simulink library "sm_car_4post_lib"  (R2021b)
settings: Solver=VariableStepAuto  StartTime=0.0  StopTime=10.0  RelTol=1e-3
values from neighbouring files (symbols this model uses):
  Init = struct    [sm_car_4post_init_data.m]
  N = 100    [sm_extr_data_cam_roller_curve.m]
  s = sin(q)    [sm_extr_data_cam_roller_curve.m]
  Vehicle = Vehicle_03    [sm_car_4post_gen_op.m]    (also in sm_car_4post_testrig_plot2testall.m)
undefined symbols (not defined in the file or in its folder): clr_upr, hp_in_f_ua, hp_in_r_ua, hp_la_out, hp_ua_out, LAc, LAf, LAr, opc_upr, radius_upr, rhs_hp, sm_car_4post_platform, smcar_param, UAc, UAf, UAr, X, Y, Z
libraries: sm_lib x234, $bdroot x71, fl_lib x24, nesl_utility x21, simulink x3
(part 2 of 11)

== system sm_car_4post_lib/Shafts CVCV ==
  CVCV : Subsystem  VariantControl=CVCV  mask(Shafts with Constant Velocity Joints){popup_leftRight=Right, drv_sha_hp_transaxle_l=Shaft.Transaxle.sTransaxle.Value, drv_sha_transax_m=Shaft.Transaxle.m.Value, drv_sha_drvsh_m=Shaft.Driveshaft.m.Value, drv_sha_axle_m=Shaft.Axle.m.Value, clr_drv_sha_hp=smcar_param.hp.clr, opc_drv_sha_hp=smcar_param.hp.opc, rad_drv_sha_hp=smcar_param.hp.rad, clr_drv_sha_jnt=smcar_param.red, opc_drv_sha_jnt=smcar_param.part.opc, rad_drv_sha_jnt=0.03, clr_drv_sha_transax=smcar_param.gray, opc_drv_sha_transax=smcar_param.part.opc, rad_drv_sha_transax=0.025, clr_drv_sha_drvsh=smcar_param.gray, opc_drv_sha_drvsh=smcar_param.part.opc, rad_drv_sha_drvsh=0.025, clr_drv_sha_axle=smcar_param.gray, opc_drv_sha_axle=smcar_param.part.opc, rad_drv_sha_axle=0.025, len_drv_sha_transax=Shaft.Transaxle.l.Value, len_drv_sha_drvsh=Shaft.Driveshaft.l.Value, len_drv_sha_axle=Shaft.Axle.l.Value}
      mask prompts: popup_leftRight "Left/Right"; drv_sha_hp_transaxle_l "Transaxle HP [xyz] (m)"; drv_sha_transax_m "Transaxle Mass (kg)"; drv_sha_drvsh_m "Driveshaft Mass (kg)"; drv_sha_axle_m "Axle Mass (kg)"; len_drv_sha_transax "Transaxle Length (m)"; len_drv_sha_drvsh "Driveshaft Length (m)"; len_drv_sha_axle "Axle Length (m)"
      mask help: Driveshaft with Constant Velocity Joints at either end.
      mask init:
      | sm_car_4post_lib_setLeftRight(gcb,'none');
      mask TypeOptions popup_leftRight: Left | Right
      mask TypeOptions drv_sha_hp_transaxle_l:
      | Transform
      | HP Transaxle/TranslationCartesianOffset
      mask TypeOptions drv_sha_transax_m: Transaxle/shaft_m
      mask TypeOptions drv_sha_drvsh_m: Driveshaft/shaft_m
      mask TypeOptions drv_sha_axle_m: Axle/shaft_m
      mask TypeOptions clr_drv_sha_hp:
      | Vis HP
      | Transaxle/GraphicDiffuseColor
      mask TypeOptions opc_drv_sha_hp:
      | Vis HP
      | Transaxle/GraphicOpacity
      mask TypeOptions rad_drv_sha_hp:
      | Vis HP
      | Transaxle/SphereRadius
      mask TypeOptions clr_drv_sha_jnt:
      | Vis
      | CV Joint
      | Inboard/GraphicDiffuseColor | Vis
      | CV Joint
      | Outboard/GraphicDiffuseColor
      mask TypeOptions opc_drv_sha_jnt:
      | Vis
      | CV Joint
      | Inboard/GraphicOpacity | Vis
      | CV Joint
      | Outboard/GraphicOpacity
      mask TypeOptions rad_drv_sha_jnt:
      | Vis
      | CV Joint
      | Inboard/SphereRadius | Vis
      | CV Joint
      | Outboard/SphereRadius
      mask TypeOptions clr_drv_sha_transax: Transaxle/clr_shaft
      mask TypeOptions opc_drv_sha_transax: Transaxle/opc_shaft
      mask TypeOptions rad_drv_sha_transax: Transaxle/rad_shaft
      mask TypeOptions clr_drv_sha_drvsh: Driveshaft/clr_shaft
      mask TypeOptions opc_drv_sha_drvsh: Driveshaft/opc_shaft
      mask TypeOptions rad_drv_sha_drvsh: Driveshaft/rad_shaft
      mask TypeOptions clr_drv_sha_axle: Axle/clr_shaft
      mask TypeOptions opc_drv_sha_axle: Axle/opc_shaft
      mask TypeOptions rad_drv_sha_axle: Axle/rad_shaft
      mask TypeOptions len_drv_sha_transax: Transaxle/len_shaft
      mask TypeOptions len_drv_sha_drvsh: Driveshaft/len_shaft
      mask TypeOptions len_drv_sha_axle: Axle/len_shaft
      mask DialogControl cont_vis_drv_sha Prompt: Visualization
      mask DialogControl text_vis_drv_sha_clr Prompt: Color [RGB]
      mask DialogControl text_vis_drv_sha_opc Prompt: Opac. (0-1)
      mask DialogControl text_vis_drv_sha_rad Prompt: Radius (m)
      mask DialogControl text_vis_drv_sha_hp Prompt: Hardpoints
      mask DialogControl text_vis_drv_sha_joints Prompt: Joints
      mask DialogControl text_vis_drv_sha_transax Prompt: Transaxle
      mask DialogControl text_vis_drv_sha_drvsh Prompt: Driveshaft
      mask DialogControl text_vis_axle_drvsh Prompt: Axle
  F : PMIOPort  Side=Right
  P : PMIOPort  Port=2  Side=Right
  B : PMIOPort  Port=3  Side=Left
  connections:
  CVCV/RConn2 -- P/RConn1
  CVCV/RConn1 -- F/RConn1
  CVCV/LConn1 -- B/RConn1

== system sm_car_4post_lib/Shafts None ==
  None : Subsystem  VariantControl=None
  F : PMIOPort  Side=Right
  P : PMIOPort  Port=2  Side=Right
  B : PMIOPort  Port=3  Side=Left
  connections:
  None/LConn1 -- B/RConn1
  None/RConn1 -- F/RConn1
  None/RConn2 -- P/RConn1

== system sm_car_4post_lib/Sine Input ==
  Clock : Clock
  Constant : Constant  Value=wave_period*num_periods+wave_delay
  Gain : Gain  Gain=wave_amplitude
  GreaterThan : RelationalOperator  Operator=<  OutDataTypeStr=boolean  RndMeth=Simplest
  Product : Product
  Ramp : simulink/Sources/Ramp  slope=2*pi/wave_period  start=wave_delay  InitialOutput=0
  Sine Wave Function : Sin  TimeSource=Use external signal  SampleTime=0
  Out1 : Outport  VectorParamsAs1DForOutWhenUnconnected=off
  wires:
  Sine Wave Function/1 -> Gain/1
  Constant/1 -> GreaterThan/2
  Clock/1 -> GreaterThan/1
  GreaterThan/1 -> Product/2
  Gain/1 -> Product/1
  Ramp/1 -> Sine Wave Function/1
  Product/1 -> Out1/1

== system sm_car_4post_lib/Spring ==
  Ctrl : Inport
  Linear : Subsystem  VariantControl=Linear  mask(Linear Spring){spr_def0=Spring.xPreload.Value, spr_k=Spring.K.Value, spr_hp_top=Spring.sTop.Value, spr_hp_bot=Spring.sBottom.Value}
      mask prompts: spr_def0 "Spr. Preload (m)"; spr_k "Spring Rate (N/m)"; spr_hp_top "HP Top [xyz] (m)"; spr_hp_bot "HP Bottom [xyz] (m)"
      mask help: Spring with linear behavior with measurements.
      mask init:
      | spr_len0 = norm(spr_hp_top-spr_hp_bot);
  R : PMIOPort  Side=Left
  C : PMIOPort  Port=2  Side=Right
  meas : Outport  VectorParamsAs1DForOutWhenUnconnected=off
  wires:
  Ctrl/1 -> Linear/1(Ctrl)
  Linear/1(meas) -> meas/1
  connections:
  Linear/RConn1 -- C/RConn1
  Linear/LConn1 -- R/RConn1

== system sm_car_4post_lib/Suspension and Steering ==
  CtrlBus : Inport
  DrvBus : Inport  Port=2
  Linkage : Subsystem  VariantControl=Linkage
  AxleL : PMIOPort  Side=Left
  Ref : PMIOPort  Port=2  Side=Right
  AxleR : PMIOPort  Port=3  Side=Right
  BrkL : PMIOPort  Port=4  Side=Left
  BrkR : PMIOPort  Port=5  Side=Right
  SprL : PMIOPort  Port=6  Side=Left
  SprR : PMIOPort  Port=7  Side=Right
  DmpL : PMIOPort  Port=8  Side=Left
  DmpR : PMIOPort  Port=9  Side=Right
  OutBus : Outport  VectorParamsAs1DForOutWhenUnconnected=off
  wires:
  CtrlBus/1 -> Linkage/1(CtrlBus)
  Linkage/1(OutBus) -> OutBus/1
  DrvBus/1 -> Linkage/2(DrvBus)
  connections:
  Linkage/LConn1 -- AxleL/RConn1
  Linkage/RConn1 -- Ref/RConn1
  Linkage/RConn4 -- SprR/RConn1
  Linkage/RConn5 -- DmpR/RConn1
  Linkage/LConn2 -- BrkL/RConn1
  Linkage/LConn3 -- SprL/RConn1
  Linkage/RConn2 -- AxleR/RConn1
  Linkage/LConn4 -- DmpL/RConn1
  Linkage/RConn3 -- BrkR/RConn1

== system sm_car_4post_lib/Utilities ==
  Camera Frames : Subsystem
      mask Display: disp('Cam')
  Cylinder Between Two Points : Subsystem  mask{hp_b=hp_la_out.*rhs_hp, hp_f=hp_ua_out.*rhs_hp, Mass=0, clr_solid=clr_upr*0+[0.2 0.4 0.6], opc_solid=opc_upr*0.5, rad_solid=radius_upr*1.5}
      mask prompts: hp_b "Hardpoint at B [xyz] (m)"; hp_f "Hardpoint at F [xyz] (m)"; Mass "Mass (kg)"; clr_solid "Color [RGB]"; opc_solid "Opacity (0-1)"; rad_solid "Radius (m)"
      mask TypeOptions Mass: Solid/Mass
      mask TypeOptions clr_solid: Solid/GraphicDiffuseColor
      mask TypeOptions opc_solid: Solid/GraphicOpacity
      mask TypeOptions rad_solid: Solid/CylinderRadius
      mask DialogControl cont_vis Prompt: Visualization
      mask Display: image(fullfile(matlabroot,'toolbox','physmod','sm','smdemos','car_4post_testrig','images','sm_car_4post_cylinder_two_points.png'))
  Primitive Bushing : Subsystem
      mask Display: image(fullfile(matlabroot,'toolbox','physmod','sm','smdemos','car_4post_testrig','images','sm_car_4post_primitive_bushing.png'));
  Primitive Gimbal : Subsystem
      mask Display: image(fullfile(matlabroot,'toolbox','physmod','sm','smdemos','car_4post_testrig','images','sm_car_4post_primitive_gimbal.png'))
  Terminator : Subsystem
  Transform Align Axis Two Points : Subsystem  mask(Transform Align Axis Two Points){hp_b=[1 1 0], hp_t=[4 5 0], popup_f_axis=+X}
      mask prompts: hp_b "Location of B [xyz] (m)"; hp_t "Target for Frame Axis [xyz] (m)"; popup_f_axis "Axis of F Frame to Aim at Target"
      mask help: Transforms a frame to aim a selected axis at a target point. Both points must be defined relative to the same reference frame.
      mask init:
      | switch popup_f_axis
      |     case 1, vec = [ 1  0  0];
      |     case 2, vec = [ 0  1  0];
      |     case 3, vec = [ 0  0  1];
      |     case 4, vec = [-1  0  0];
      |     case 5, vec = [ 0 -1  0];
      |     case 6, vec = [ 0  0 -1];
      | end
      | 
      | uvec_bt = (hp_t-hp_b)/norm(hp_t-hp_b);
      | rotaxis = cross(vec,uvec_bt);
      | 
      | if (norm(rotaxis)==0)
      |     if (uvec_bt==0)            % hps collocated
      |         rotangle = 0; 
      |     elseif ((uvec_bt+vec)==0)  % vectors antiparallel    
      |         rotangle = pi;
      |         rotaxis = circshift(vec,1);
      |     else                       % vectors parallel
      |         rotangle = 0;          
      |     end
      | else
      |     rotangle = acos(dot(vec,uvec_bt));
      |     %rotangle = acos(dot(vec,(hp_t-hp_b)/norm((hp_t-hp_b))))
      | end
      mask TypeOptions popup_f_axis: +X | +Y | +Z | -X | -Y | -Z
      mask Display: image(fullfile(matlabroot,'toolbox','physmod','sm','smdemos','car_4post_testrig','images','sm_car_4post_transform_align_axis_two_points.png'))
  Universal Two HP : Subsystem  mask{popup_leftRight=Left, hp_f=hp_in_f_ua, hp_r=hp_in_r_ua}
      mask prompts: popup_leftRight "Left/Right"; hp_f "HP Front [xyz] (m)"; hp_r "HP Rear [xyz] (m)"
      mask init:
      | if(popup_leftRight == 1)
      |     rhs_y = 1;
      | elseif(popup_leftRight == 2)
      |     rhs_y = -1;
      | end
      | 
      | rhs_hp = [1 rhs_y 1];
      mask TypeOptions popup_leftRight: Left | Right
      mask Display: image(fullfile(matlabroot,'toolbox','physmod','sm','smdemos','car_4post_testrig','images','sm_car_4post_variant_universal.png'));

== system sm_car_4post_lib/Wheel ==
  RdBus : Inport
  Post : Subsystem  VariantControl=MFEval  mask{popup_leftRight=Left, platform=sm_car_4post_platform, clr_tyre=[0.5 0.5 0.5], opc_tyre=1, clr_rim=[0.8 0.8 0.8], opc_rim=0.5}
      mask prompts: popup_leftRight "Left/Right"; platform "Platform Data"
      mask init:
      | if(popup_leftRight == 1)
      |     set_param([gcb '/Tire Body'],'popup_leftRight','Left');
      |     rhs_whl = [1 1 1];
      | elseif(popup_leftRight == 2)
      |     set_param([gcb '/Tire Body'],'popup_leftRight','Right');
      |     rhs_whl = [1 -1 1];
      | end
      mask TypeOptions popup_leftRight: Left | Right
      mask TypeOptions clr_tyre: Tire Body/clr_tyre
      mask TypeOptions opc_tyre: Tire Body/opc_tyre
      mask TypeOptions clr_rim: Tire Body/clr_rim
      mask TypeOptions opc_rim: Tire Body/opc_rim
      mask DialogControl cont_tire_mfeval Prompt: Platform
      mask DialogControl cont_vis Prompt: Visualization
      mask DialogControl text_vis_clr Prompt: Color [RGB]
      mask DialogControl text_vis_opc Prompt: Opacity (0-1)
      mask DialogControl text_tyre Prompt: Tyre
      mask DialogControl text_rim Prompt: Rim
  B : PMIOPort  Side=Right
  C : PMIOPort  Port=2  Side=Left
  Out : Outport  VectorParamsAs1DForOutWhenUnconnected=off
  wires:
  RdBus/1 -> Post/1(RdBus)
  Post/1(Out) -> Out/1
  connections:
  Post/LConn1 -- C/RConn1
  Post/RConn1 -- B/RConn1

== system sm_car_4post_lib/Damper/Linear ==
  note: Sensing
  Ctrl : Inport
  Bumpstop : fl_lib/Mechanical/Translational Elements/Translational Hard Stop  upper_bnd=bs_lim_upper m  lower_bnd=bs_lim_lower m  stiff_up=bs_k_upper N/m  stiff_low=bs_k_lower N/m  D_up=bs_b_upper N/(m/s)  D_low=bs_b_lower N/(m/s)  model=1  transition=bs_region m  v_specify=off  v_priority=None  v=0 m/s  v_nominal_specify=off  v_nominal_unit=m/s  v_nominal_value=1  f_specify=off  f_priority=None  f=0 N  f_nominal_specify=off  f_nominal_unit=N  f_nominal_value=1  x_specify=off  x_priority=High  x=0 m  x_nominal_specify=off  x_nominal_unit=m  x_nominal_value=1
  Damper : fl_lib/Mechanical/Translational Elements/Translational Damper  D=dam_b N/(m/s)  v_specify=off  v_priority=None  v=0 m/s  v_nominal_specify=off  v_nominal_unit=m/s  v_nominal_value=1  f_specify=off  f_priority=None  f=0 N  f_nominal_specify=off  f_nominal_unit=N  f_nominal_value=1
  Force Bumpstop : fl_lib/Mechanical/Mechanical Sensors/Ideal Force Sensor
  Force Damper : fl_lib/Mechanical/Mechanical Sensors/Ideal Force Sensor
  Motion Damper : fl_lib/Mechanical/Mechanical Sensors/Ideal Translational Motion Sensor  offset=dam_x0 m
  PS-Simulink Converter : nesl_utility/PS-Simulink Converter  PhysicalDomain=network_engine_domain  SubClassName=ps_output  LeftPortType=input  RightPortType=output  PseudoPeriodic=off  Frequencies=[]  Unit=N  AffineConversion=off
      settings: SourceProductBaseCode=PW,SS
  PS-Simulink Converter1 : nesl_utility/PS-Simulink Converter  PhysicalDomain=network_engine_domain  SubClassName=ps_output  LeftPortType=input  RightPortType=output  PseudoPeriodic=off  Frequencies=[]  Unit=N  AffineConversion=off
      settings: SourceProductBaseCode=PW,SS
  PS-Simulink Converter2 : nesl_utility/PS-Simulink Converter  PhysicalDomain=network_engine_domain  SubClassName=ps_output  LeftPortType=input  RightPortType=output  PseudoPeriodic=off  Frequencies=[]  Unit=m/s  AffineConversion=off
      settings: SourceProductBaseCode=PW,SS
  PS-Simulink Converter3 : nesl_utility/PS-Simulink Converter  PhysicalDomain=network_engine_domain  SubClassName=ps_output  LeftPortType=input  RightPortType=output  PseudoPeriodic=off  Frequencies=[]  Unit=m  AffineConversion=off
      settings: SourceProductBaseCode=PW,SS
  Terminator : Terminator
  R : PMIOPort  Side=Left
  C : PMIOPort  Port=2  Side=Right
  Out Bus Element : Outport  VectorParamsAs1DForOutWhenUnconnected=off  PortName=meas  Element=FDamper
  Out Bus Element1 : Outport  VectorParamsAs1DForOutWhenUnconnected=off  PortName=meas  Element=FBumpstop
  Out Bus Element2 : Outport  VectorParamsAs1DForOutWhenUnconnected=off  PortName=meas  Element=xDamper
  Out Bus Element3 : Outport  VectorParamsAs1DForOutWhenUnconnected=off  PortName=meas  Element=vDamper
  wires:
  PS-Simulink Converter1/1 -> Out Bus Element1/1
  PS-Simulink Converter3/1 -> Out Bus Element2/1
  PS-Simulink Converter2/1 -> Out Bus Element3/1
  PS-Simulink Converter/1 -> Out Bus Element/1
  Ctrl/1 -> Terminator/1
  connections:
  R/RConn1 -- Motion Damper/LConn1 -- Bumpstop/LConn1 -- Damper/LConn1
  Force Damper/RConn1 -- Damper/RConn1
  Force Bumpstop/RConn1 -- Bumpstop/RConn1
  PS-Simulink Converter/LConn1 -- Force Damper/RConn2
  PS-Simulink Converter3/LConn1 -- Motion Damper/RConn3
  PS-Simulink Converter1/LConn1 -- Force Bumpstop/RConn2
  PS-Simulink Converter2/LConn1 -- Motion Damper/RConn2
  Force Damper/LConn1 -- C/RConn1 -- Force Bumpstop/LConn1 -- Motion Damper/RConn1
